simulink model "SRSModeState"  (R2018b)
settings: Solver=FixedStepDiscrete  StartTime=0.0  StopTime=10.0  FixedStep=0.01  RelTol=1e-3
undefined symbols (not defined in the file or in its folder): KeSMSuMdNums_Val, MdTp1, SrcReqTp1, SRSconvertArray_Val
libraries: RspLib x32
settings Model: Creator=sn2xws  LastModifiedBy=sn2xws
settings DataIOCC: SaveFormat=StructureWithTime
settings OptimizationCC: DefaultParameterBehavior=Inlined  EnhancedBackFolding=on  PassReuseOutputArgsAs=Individual arguments  ZeroExternalMemoryAtStartup=off  ZeroInternalMemoryAtStartup=off  OptimizeBlockOrder=speed  DifferentSizesBufferReuse=on  OptimizationCustomize=off
settings DebuggingCC: ParameterTunabilityLossMsg=error
settings ModelReferenceCC: ModelReferenceNumInstancesAllowed=Single
settings SFSimCC: MATLABDynamicMemAlloc=off
settings RTWCC: SystemTargetFile=autosar.tlc  GenCodeOnly=on  TemplateMakefile=ert_default_tmf  Description=AUTOSAR  GenerateReport=on  IncludeHyperlinkInReport=on  LaunchReport=on  GenerateTraceInfo=on  GenerateTraceReport=on  GenerateTraceReportSl=on  GenerateTraceReportSf=on  GenerateTraceReportEml=on  GenerateCodeMetricsReport=on
settings CodeAppCC: ForceParamTrailComments=on  IgnoreCustomStorageClasses=off  OperatorAnnotations=on  SimulinkDataObjDesc=on  SFDataObjDesc=on  InsertBlockDesc=on
settings STFCustomTargetCC: TargetLangStandard=C99 (ISO)  MultiwordLength=256  ParMdlRefBuildCompliant=on  CompOptLevelCompliant=on  IncludeMdlTerminateFcn=off  CombineOutputUpdateFcns=on  SuppressErrorStatus=on  ERTCustomFileBanners=on  SupportNonFinite=off  SupportComplex=off  SupportContinuousTime=off  SupportNonInlinedSFcns=off  RemoveResetFunc=on  MATLABClassNameForMDSCustomization=Simulink.SoftwareTarget.ERTCustomization  AutosarCompliant=on  UseToolchainInfoCompliant=on  LookupTableObjectStructAxisOrder=2,1,3,4,...  LUTObjectStructOrderEvenSpacing=Size,Table,Breakpoints  SystemTargetFile=autosar.tlc
settings ERTTargetCC: TargetLangStandard=C99 (ISO)  ConcurrentExecutionCompliant=off  IncludeMdlTerminateFcn=off  SuppressErrorStatus=on  SupportNonFinite=off  SupportComplex=off  ModelStepFunctionPrototypeControlCompliant=off  CPPClassGenCompliant=off  AutosarCompliant=on  LookupTableObjectStructAxisOrder=2,1,3,4,...  LUTObjectStructOrderEvenSpacing=Size,Table,Breakpoints  InlinedParameterPlacement=NonHierarchical  ERTCustomFileTemplate=example_file_process.tlc  ERTFilePackagingFormat=Compact

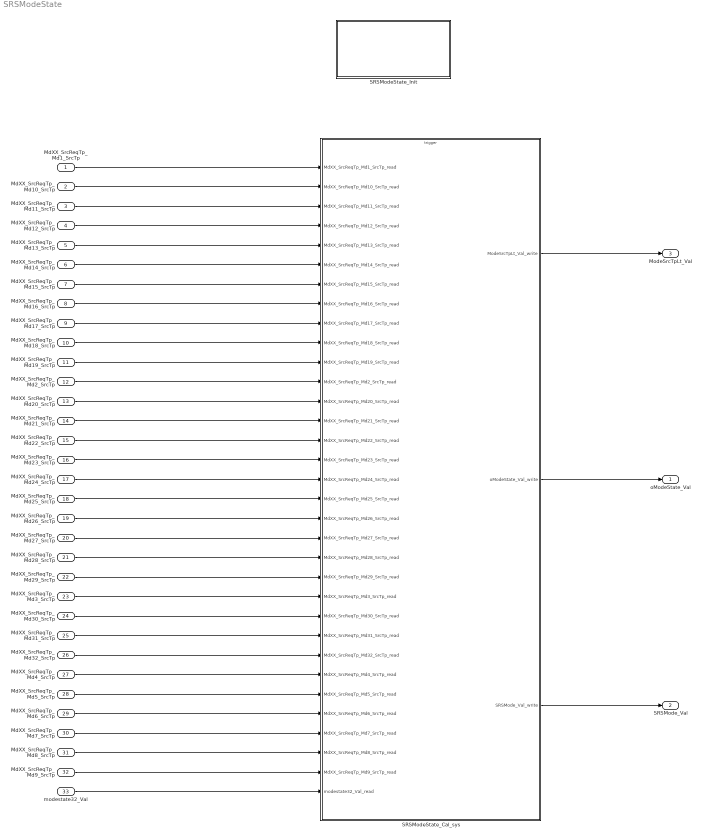
== system SRSModeState ==
  MdXX_SrcReqTp_Md1_SrcTp : Inport  OutDataTypeStr=Enum: SrcReqTp1  PortDimensions=1
  MdXX_SrcReqTp_Md10_SrcTp : Inport  Port=2  OutDataTypeStr=Enum: SrcReqTp1  PortDimensions=1
  MdXX_SrcReqTp_Md11_SrcTp : Inport  Port=3  OutDataTypeStr=Enum: SrcReqTp1  PortDimensions=1
  MdXX_SrcReqTp_Md12_SrcTp : Inport  Port=4  OutDataTypeStr=Enum: SrcReqTp1  PortDimensions=1
  MdXX_SrcReqTp_Md13_SrcTp : Inport  Port=5  OutDataTypeStr=Enum: SrcReqTp1  PortDimensions=1
  MdXX_SrcReqTp_Md14_SrcTp : Inport  Port=6  OutDataTypeStr=Enum: SrcReqTp1  PortDimensions=1
  MdXX_SrcReqTp_Md15_SrcTp : Inport  Port=7  OutDataTypeStr=Enum: SrcReqTp1  PortDimensions=1
  MdXX_SrcReqTp_Md16_SrcTp : Inport  Port=8  OutDataTypeStr=Enum: SrcReqTp1  PortDimensions=1
  MdXX_SrcReqTp_Md17_SrcTp : Inport  Port=9  OutDataTypeStr=Enum: SrcReqTp1  PortDimensions=1
  MdXX_SrcReqTp_Md18_SrcTp : Inport  Port=10  OutDataTypeStr=Enum: SrcReqTp1  PortDimensions=1
  MdXX_SrcReqTp_Md19_SrcTp : Inport  Port=11  OutDataTypeStr=Enum: SrcReqTp1  PortDimensions=1
  MdXX_SrcReqTp_Md2_SrcTp : Inport  Port=12  OutDataTypeStr=Enum: SrcReqTp1  PortDimensions=1
  MdXX_SrcReqTp_Md20_SrcTp : Inport  Port=13  OutDataTypeStr=Enum: SrcReqTp1  PortDimensions=1
  MdXX_SrcReqTp_Md21_SrcTp : Inport  Port=14  OutDataTypeStr=Enum: SrcReqTp1  PortDimensions=1
  MdXX_SrcReqTp_Md22_SrcTp : Inport  Port=15  OutDataTypeStr=Enum: SrcReqTp1  PortDimensions=1
  MdXX_SrcReqTp_Md23_SrcTp : Inport  Port=16  OutDataTypeStr=Enum: SrcReqTp1  PortDimensions=1
  MdXX_SrcReqTp_Md24_SrcTp : Inport  Port=17  OutDataTypeStr=Enum: SrcReqTp1  PortDimensions=1
  MdXX_SrcReqTp_Md25_SrcTp : Inport  Port=18  OutDataTypeStr=Enum: SrcReqTp1  PortDimensions=1
  MdXX_SrcReqTp_Md26_SrcTp : Inport  Port=19  OutDataTypeStr=Enum: SrcReqTp1  PortDimensions=1
  MdXX_SrcReqTp_Md27_SrcTp : Inport  Port=20  OutDataTypeStr=Enum: SrcReqTp1  PortDimensions=1
  MdXX_SrcReqTp_Md28_SrcTp : Inport  Port=21  OutDataTypeStr=Enum: SrcReqTp1  PortDimensions=1
  MdXX_SrcReqTp_Md29_SrcTp : Inport  Port=22  OutDataTypeStr=Enum: SrcReqTp1  PortDimensions=1
  MdXX_SrcReqTp_Md3_SrcTp : Inport  Port=23  OutDataTypeStr=Enum: SrcReqTp1  PortDimensions=1
  MdXX_SrcReqTp_Md30_SrcTp : Inport  Port=24  OutDataTypeStr=Enum: SrcReqTp1  PortDimensions=1
  MdXX_SrcReqTp_Md31_SrcTp : Inport  Port=25  OutDataTypeStr=Enum: SrcReqTp1  PortDimensions=1
  MdXX_SrcReqTp_Md32_SrcTp : Inport  Port=26  OutDataTypeStr=Enum: SrcReqTp1  PortDimensions=1
  MdXX_SrcReqTp_Md4_SrcTp : Inport  Port=27  OutDataTypeStr=Enum: SrcReqTp1  PortDimensions=1
  MdXX_SrcReqTp_Md5_SrcTp : Inport  Port=28  OutDataTypeStr=Enum: SrcReqTp1  PortDimensions=1
  MdXX_SrcReqTp_Md6_SrcTp : Inport  Port=29  OutDataTypeStr=Enum: SrcReqTp1  PortDimensions=1
  MdXX_SrcReqTp_Md7_SrcTp : Inport  Port=30  OutDataTypeStr=Enum: SrcReqTp1  PortDimensions=1
  MdXX_SrcReqTp_Md8_SrcTp : Inport  Port=31  OutDataTypeStr=Enum: SrcReqTp1  PortDimensions=1
  MdXX_SrcReqTp_Md9_SrcTp : Inport  Port=32  OutDataTypeStr=Enum: SrcReqTp1  PortDimensions=1
  modestate32_Val : Inport  Port=33  OutDataTypeStr=uint32  PortDimensions=1
  SRSModeState_Cal_sys : Subsystem
  SRSModeState_Init : Subsystem
  oModeState_Val : Outport  OutDataTypeStr=Enum: MdTp1  PortDimensions=1
  SRSMode_Val : Outport  Port=2  OutDataTypeStr=Enum: SRSCurMode2  PortDimensions=1
  ModeSrcTpLt_Val : Outport  Port=3  OutDataTypeStr=Enum: SrcReqTp1  PortDimensions=1
  wires:
  MdXX_SrcReqTp_Md1_SrcTp/1 -> SRSModeState_Cal_sys/1(MdXX_SrcReqTp_Md1_SrcTp_read)
  MdXX_SrcReqTp_Md10_SrcTp/1 -> SRSModeState_Cal_sys/2(MdXX_SrcReqTp_Md10_SrcTp_read)
  MdXX_SrcReqTp_Md11_SrcTp/1 -> SRSModeState_Cal_sys/3(MdXX_SrcReqTp_Md11_SrcTp_read)
  MdXX_SrcReqTp_Md12_SrcTp/1 -> SRSModeState_Cal_sys/4(MdXX_SrcReqTp_Md12_SrcTp_read)
  MdXX_SrcReqTp_Md13_SrcTp/1 -> SRSModeState_Cal_sys/5(MdXX_SrcReqTp_Md13_SrcTp_read)
  MdXX_SrcReqTp_Md14_SrcTp/1 -> SRSModeState_Cal_sys/6(MdXX_SrcReqTp_Md14_SrcTp_read)
  MdXX_SrcReqTp_Md15_SrcTp/1 -> SRSModeState_Cal_sys/7(MdXX_SrcReqTp_Md15_SrcTp_read)
  MdXX_SrcReqTp_Md16_SrcTp/1 -> SRSModeState_Cal_sys/8(MdXX_SrcReqTp_Md16_SrcTp_read)
  MdXX_SrcReqTp_Md17_SrcTp/1 -> SRSModeState_Cal_sys/9(MdXX_SrcReqTp_Md17_SrcTp_read)
  MdXX_SrcReqTp_Md18_SrcTp/1 -> SRSModeState_Cal_sys/10(MdXX_SrcReqTp_Md18_SrcTp_read)
  MdXX_SrcReqTp_Md19_SrcTp/1 -> SRSModeState_Cal_sys/11(MdXX_SrcReqTp_Md19_SrcTp_read)
  MdXX_SrcReqTp_Md2_SrcTp/1 -> SRSModeState_Cal_sys/12(MdXX_SrcReqTp_Md2_SrcTp_read)
  MdXX_SrcReqTp_Md20_SrcTp/1 -> SRSModeState_Cal_sys/13(MdXX_SrcReqTp_Md20_SrcTp_read)
  MdXX_SrcReqTp_Md21_SrcTp/1 -> SRSModeState_Cal_sys/14(MdXX_SrcReqTp_Md21_SrcTp_read)
  MdXX_SrcReqTp_Md22_SrcTp/1 -> SRSModeState_Cal_sys/15(MdXX_SrcReqTp_Md22_SrcTp_read)
  MdXX_SrcReqTp_Md23_SrcTp/1 -> SRSModeState_Cal_sys/16(MdXX_SrcReqTp_Md23_SrcTp_read)
  MdXX_SrcReqTp_Md24_SrcTp/1 -> SRSModeState_Cal_sys/17(MdXX_SrcReqTp_Md24_SrcTp_read)
  MdXX_SrcReqTp_Md25_SrcTp/1 -> SRSModeState_Cal_sys/18(MdXX_SrcReqTp_Md25_SrcTp_read)
  MdXX_SrcReqTp_Md26_SrcTp/1 -> SRSModeState_Cal_sys/19(MdXX_SrcReqTp_Md26_SrcTp_read)
  MdXX_SrcReqTp_Md27_SrcTp/1 -> SRSModeState_Cal_sys/20(MdXX_SrcReqTp_Md27_SrcTp_read)
  MdXX_SrcReqTp_Md28_SrcTp/1 -> SRSModeState_Cal_sys/21(MdXX_SrcReqTp_Md28_SrcTp_read)
  MdXX_SrcReqTp_Md29_SrcTp/1 -> SRSModeState_Cal_sys/22(MdXX_SrcReqTp_Md29_SrcTp_read)
  MdXX_SrcReqTp_Md3_SrcTp/1 -> SRSModeState_Cal_sys/23(MdXX_SrcReqTp_Md3_SrcTp_read)
  MdXX_SrcReqTp_Md30_SrcTp/1 -> SRSModeState_Cal_sys/24(MdXX_SrcReqTp_Md30_SrcTp_read)
  MdXX_SrcReqTp_Md31_SrcTp/1 -> SRSModeState_Cal_sys/25(MdXX_SrcReqTp_Md31_SrcTp_read)
  MdXX_SrcReqTp_Md32_SrcTp/1 -> SRSModeState_Cal_sys/26(MdXX_SrcReqTp_Md32_SrcTp_read)
  MdXX_SrcReqTp_Md4_SrcTp/1 -> SRSModeState_Cal_sys/27(MdXX_SrcReqTp_Md4_SrcTp_read)
  MdXX_SrcReqTp_Md5_SrcTp/1 -> SRSModeState_Cal_sys/28(MdXX_SrcReqTp_Md5_SrcTp_read)
  MdXX_SrcReqTp_Md6_SrcTp/1 -> SRSModeState_Cal_sys/29(MdXX_SrcReqTp_Md6_SrcTp_read)
  MdXX_SrcReqTp_Md7_SrcTp/1 -> SRSModeState_Cal_sys/30(MdXX_SrcReqTp_Md7_SrcTp_read)
  MdXX_SrcReqTp_Md8_SrcTp/1 -> SRSModeState_Cal_sys/31(MdXX_SrcReqTp_Md8_SrcTp_read)
  MdXX_SrcReqTp_Md9_SrcTp/1 -> SRSModeState_Cal_sys/32(MdXX_SrcReqTp_Md9_SrcTp_read)
  modestate32_Val/1 -> SRSModeState_Cal_sys/33(modestate32_Val_read)
  SRSModeState_Cal_sys/1(ModeSrcTpLt_Val_write) -> ModeSrcTpLt_Val/1
  SRSModeState_Cal_sys/3(SRSMode_Val_write) -> SRSMode_Val/1
  SRSModeState_Cal_sys/2(oModeState_Val_write) -> oModeState_Val/1

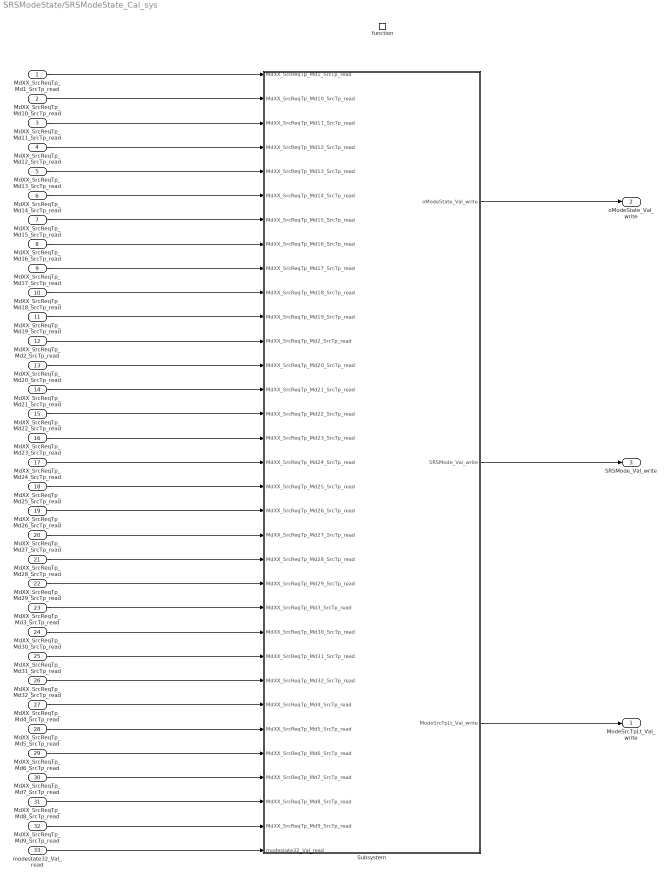
== system SRSModeState/SRSModeState_Cal_sys ==
  MdXX_SrcReqTp_Md1_SrcTp_read : Inport
  MdXX_SrcReqTp_Md10_SrcTp_read : Inport  Port=2
  MdXX_SrcReqTp_Md11_SrcTp_read : Inport  Port=3
  MdXX_SrcReqTp_Md12_SrcTp_read : Inport  Port=4
  MdXX_SrcReqTp_Md13_SrcTp_read : Inport  Port=5
  MdXX_SrcReqTp_Md14_SrcTp_read : Inport  Port=6
  MdXX_SrcReqTp_Md15_SrcTp_read : Inport  Port=7
  MdXX_SrcReqTp_Md16_SrcTp_read : Inport  Port=8
  MdXX_SrcReqTp_Md17_SrcTp_read : Inport  Port=9
  MdXX_SrcReqTp_Md18_SrcTp_read : Inport  Port=10
  MdXX_SrcReqTp_Md19_SrcTp_read : Inport  Port=11
  MdXX_SrcReqTp_Md2_SrcTp_read : Inport  Port=12
  MdXX_SrcReqTp_Md20_SrcTp_read : Inport  Port=13
  MdXX_SrcReqTp_Md21_SrcTp_read : Inport  Port=14
  MdXX_SrcReqTp_Md22_SrcTp_read : Inport  Port=15
  MdXX_SrcReqTp_Md23_SrcTp_read : Inport  Port=16
  MdXX_SrcReqTp_Md24_SrcTp_read : Inport  Port=17
  MdXX_SrcReqTp_Md25_SrcTp_read : Inport  Port=18
  MdXX_SrcReqTp_Md26_SrcTp_read : Inport  Port=19
  MdXX_SrcReqTp_Md27_SrcTp_read : Inport  Port=20
  MdXX_SrcReqTp_Md28_SrcTp_read : Inport  Port=21
  MdXX_SrcReqTp_Md29_SrcTp_read : Inport  Port=22
  MdXX_SrcReqTp_Md3_SrcTp_read : Inport  Port=23
  MdXX_SrcReqTp_Md30_SrcTp_read : Inport  Port=24
  MdXX_SrcReqTp_Md31_SrcTp_read : Inport  Port=25
  MdXX_SrcReqTp_Md32_SrcTp_read : Inport  Port=26
  MdXX_SrcReqTp_Md4_SrcTp_read : Inport  Port=27
  MdXX_SrcReqTp_Md5_SrcTp_read : Inport  Port=28
  MdXX_SrcReqTp_Md6_SrcTp_read : Inport  Port=29
  MdXX_SrcReqTp_Md7_SrcTp_read : Inport  Port=30
  MdXX_SrcReqTp_Md8_SrcTp_read : Inport  Port=31
  MdXX_SrcReqTp_Md9_SrcTp_read : Inport  Port=32
  modestate32_Val_read : Inport  Port=33
  function : TriggerPort  TriggerType=function-call  IsSimulinkFunction=on  FunctionName=SRSModeState_Cal  VariantControl=(inherit)
  Subsystem : Subsystem
  ModeSrcTpLt_Val_write : Outport
      settings: EnsureOutportIsVirtual=on
  oModeState_Val_write : Outport  Port=2
      settings: EnsureOutportIsVirtual=on
  SRSMode_Val_write : Outport  Port=3
      settings: EnsureOutportIsVirtual=on
  wires:
  MdXX_SrcReqTp_Md12_SrcTp_read/1 -> Subsystem/4(MdXX_SrcReqTp_Md12_SrcTp_read)
  MdXX_SrcReqTp_Md13_SrcTp_read/1 -> Subsystem/5(MdXX_SrcReqTp_Md13_SrcTp_read)
  MdXX_SrcReqTp_Md1_SrcTp_read/1 -> Subsystem/1(MdXX_SrcReqTp_Md1_SrcTp_read)
  MdXX_SrcReqTp_Md10_SrcTp_read/1 -> Subsystem/2(MdXX_SrcReqTp_Md10_SrcTp_read)
  MdXX_SrcReqTp_Md11_SrcTp_read/1 -> Subsystem/3(MdXX_SrcReqTp_Md11_SrcTp_read)
  MdXX_SrcReqTp_Md14_SrcTp_read/1 -> Subsystem/6(MdXX_SrcReqTp_Md14_SrcTp_read)
  MdXX_SrcReqTp_Md15_SrcTp_read/1 -> Subsystem/7(MdXX_SrcReqTp_Md15_SrcTp_read)
  MdXX_SrcReqTp_Md16_SrcTp_read/1 -> Subsystem/8(MdXX_SrcReqTp_Md16_SrcTp_read)
  MdXX_SrcReqTp_Md17_SrcTp_read/1 -> Subsystem/9(MdXX_SrcReqTp_Md17_SrcTp_read)
  MdXX_SrcReqTp_Md18_SrcTp_read/1 -> Subsystem/10(MdXX_SrcReqTp_Md18_SrcTp_read)
  MdXX_SrcReqTp_Md19_SrcTp_read/1 -> Subsystem/11(MdXX_SrcReqTp_Md19_SrcTp_read)
  MdXX_SrcReqTp_Md2_SrcTp_read/1 -> Subsystem/12(MdXX_SrcReqTp_Md2_SrcTp_read)
  MdXX_SrcReqTp_Md20_SrcTp_read/1 -> Subsystem/13(MdXX_SrcReqTp_Md20_SrcTp_read)
  MdXX_SrcReqTp_Md21_SrcTp_read/1 -> Subsystem/14(MdXX_SrcReqTp_Md21_SrcTp_read)
  MdXX_SrcReqTp_Md22_SrcTp_read/1 -> Subsystem/15(MdXX_SrcReqTp_Md22_SrcTp_read)
  MdXX_SrcReqTp_Md23_SrcTp_read/1 -> Subsystem/16(MdXX_SrcReqTp_Md23_SrcTp_read)
  MdXX_SrcReqTp_Md24_SrcTp_read/1 -> Subsystem/17(MdXX_SrcReqTp_Md24_SrcTp_read)
  MdXX_SrcReqTp_Md25_SrcTp_read/1 -> Subsystem/18(MdXX_SrcReqTp_Md25_SrcTp_read)
  MdXX_SrcReqTp_Md26_SrcTp_read/1 -> Subsystem/19(MdXX_SrcReqTp_Md26_SrcTp_read)
  MdXX_SrcReqTp_Md27_SrcTp_read/1 -> Subsystem/20(MdXX_SrcReqTp_Md27_SrcTp_read)
  MdXX_SrcReqTp_Md28_SrcTp_read/1 -> Subsystem/21(MdXX_SrcReqTp_Md28_SrcTp_read)
  MdXX_SrcReqTp_Md29_SrcTp_read/1 -> Subsystem/22(MdXX_SrcReqTp_Md29_SrcTp_read)
  MdXX_SrcReqTp_Md3_SrcTp_read/1 -> Subsystem/23(MdXX_SrcReqTp_Md3_SrcTp_read)
  MdXX_SrcReqTp_Md30_SrcTp_read/1 -> Subsystem/24(MdXX_SrcReqTp_Md30_SrcTp_read)
  MdXX_SrcReqTp_Md31_SrcTp_read/1 -> Subsystem/25(MdXX_SrcReqTp_Md31_SrcTp_read)
  MdXX_SrcReqTp_Md32_SrcTp_read/1 -> Subsystem/26(MdXX_SrcReqTp_Md32_SrcTp_read)
  MdXX_SrcReqTp_Md4_SrcTp_read/1 -> Subsystem/27(MdXX_SrcReqTp_Md4_SrcTp_read)
  MdXX_SrcReqTp_Md5_SrcTp_read/1 -> Subsystem/28(MdXX_SrcReqTp_Md5_SrcTp_read)
  MdXX_SrcReqTp_Md6_SrcTp_read/1 -> Subsystem/29(MdXX_SrcReqTp_Md6_SrcTp_read)
  MdXX_SrcReqTp_Md7_SrcTp_read/1 -> Subsystem/30(MdXX_SrcReqTp_Md7_SrcTp_read)
  MdXX_SrcReqTp_Md8_SrcTp_read/1 -> Subsystem/31(MdXX_SrcReqTp_Md8_SrcTp_read)
  MdXX_SrcReqTp_Md9_SrcTp_read/1 -> Subsystem/32(MdXX_SrcReqTp_Md9_SrcTp_read)
  modestate32_Val_read/1 -> Subsystem/33(modestate32_Val_read)
  Subsystem/1(oModeState_Val_write) -> oModeState_Val_write/1
  Subsystem/2(SRSMode_Val_write) -> SRSMode_Val_write/1
  Subsystem/3(ModeSrcTpLt_Val_write) -> ModeSrcTpLt_Val_write/1

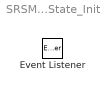
== system SRSModeState/SRSModeState_Init ==
  Event Listener : EventListener  EventName=reset

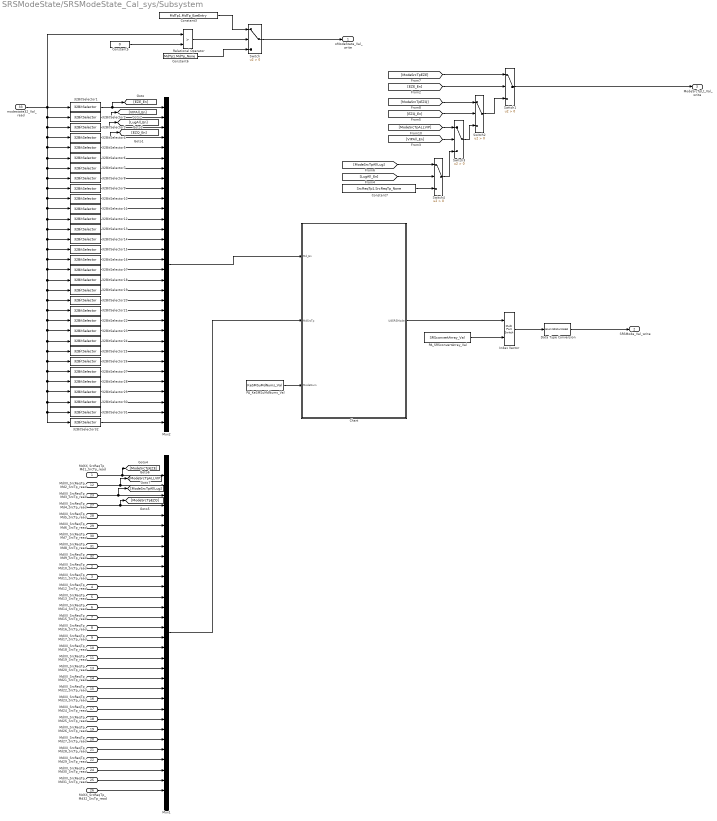
== system SRSModeState/SRSModeState_Cal_sys/Subsystem ==
  MdXX_SrcReqTp_Md1_SrcTp_read : Inport
  MdXX_SrcReqTp_Md10_SrcTp_read : Inport  Port=2
  MdXX_SrcReqTp_Md11_SrcTp_read : Inport  Port=3
  MdXX_SrcReqTp_Md12_SrcTp_read : Inport  Port=4
  MdXX_SrcReqTp_Md13_SrcTp_read : Inport  Port=5
  MdXX_SrcReqTp_Md14_SrcTp_read : Inport  Port=6
  MdXX_SrcReqTp_Md15_SrcTp_read : Inport  Port=7
  MdXX_SrcReqTp_Md16_SrcTp_read : Inport  Port=8
  MdXX_SrcReqTp_Md17_SrcTp_read : Inport  Port=9
  MdXX_SrcReqTp_Md18_SrcTp_read : Inport  Port=10
  MdXX_SrcReqTp_Md19_SrcTp_read : Inport  Port=11
  MdXX_SrcReqTp_Md2_SrcTp_read : Inport  Port=12
  MdXX_SrcReqTp_Md20_SrcTp_read : Inport  Port=13
  MdXX_SrcReqTp_Md21_SrcTp_read : Inport  Port=14
  MdXX_SrcReqTp_Md22_SrcTp_read : Inport  Port=15
  MdXX_SrcReqTp_Md23_SrcTp_read : Inport  Port=16
  MdXX_SrcReqTp_Md24_SrcTp_read : Inport  Port=17
  MdXX_SrcReqTp_Md25_SrcTp_read : Inport  Port=18
  MdXX_SrcReqTp_Md26_SrcTp_read : Inport  Port=19
  MdXX_SrcReqTp_Md27_SrcTp_read : Inport  Port=20
  MdXX_SrcReqTp_Md28_SrcTp_read : Inport  Port=21
  MdXX_SrcReqTp_Md29_SrcTp_read : Inport  Port=22
  MdXX_SrcReqTp_Md3_SrcTp_read : Inport  Port=23
  MdXX_SrcReqTp_Md30_SrcTp_read : Inport  Port=24
  MdXX_SrcReqTp_Md31_SrcTp_read : Inport  Port=25
  MdXX_SrcReqTp_Md32_SrcTp_read : Inport  Port=26
  MdXX_SrcReqTp_Md4_SrcTp_read : Inport  Port=27
  MdXX_SrcReqTp_Md5_SrcTp_read : Inport  Port=28
  MdXX_SrcReqTp_Md6_SrcTp_read : Inport  Port=29
  MdXX_SrcReqTp_Md7_SrcTp_read : Inport  Port=30
  MdXX_SrcReqTp_Md8_SrcTp_read : Inport  Port=31
  MdXX_SrcReqTp_Md9_SrcTp_read : Inport  Port=32
  modestate32_Val_read : Inport  Port=33
  32BitSelector1 : RspLib/32BitSelector  BitNum=0
  32BitSelector10 : RspLib/32BitSelector  BitNum=9
  32BitSelector11 : RspLib/32BitSelector  BitNum=10
  32BitSelector12 : RspLib/32BitSelector  BitNum=11
  32BitSelector13 : RspLib/32BitSelector  BitNum=12
  32BitSelector14 : RspLib/32BitSelector  BitNum=13
  32BitSelector15 : RspLib/32BitSelector  BitNum=14
  32BitSelector16 : RspLib/32BitSelector  BitNum=15
  32BitSelector17 : RspLib/32BitSelector  BitNum=16
  32BitSelector18 : RspLib/32BitSelector  BitNum=17
  32BitSelector19 : RspLib/32BitSelector  BitNum=18
  32BitSelector2 : RspLib/32BitSelector  BitNum=1
  32BitSelector20 : RspLib/32BitSelector  BitNum=19
  32BitSelector21 : RspLib/32BitSelector  BitNum=20
  32BitSelector22 : RspLib/32BitSelector  BitNum=21
  32BitSelector23 : RspLib/32BitSelector  BitNum=22
  32BitSelector24 : RspLib/32BitSelector  BitNum=23
  32BitSelector25 : RspLib/32BitSelector  BitNum=24
  32BitSelector26 : RspLib/32BitSelector  BitNum=25
  32BitSelector27 : RspLib/32BitSelector  BitNum=26
  32BitSelector28 : RspLib/32BitSelector  BitNum=27
  32BitSelector29 : RspLib/32BitSelector  BitNum=28
  32BitSelector3 : RspLib/32BitSelector  BitNum=2
  32BitSelector30 : RspLib/32BitSelector  BitNum=29
  32BitSelector31 : RspLib/32BitSelector  BitNum=30
  32BitSelector32 : RspLib/32BitSelector  BitNum=31
  32BitSelector4 : RspLib/32BitSelector  BitNum=3
  32BitSelector5 : RspLib/32BitSelector  BitNum=4
  32BitSelector6 : RspLib/32BitSelector  BitNum=5
  32BitSelector7 : RspLib/32BitSelector  BitNum=6
  32BitSelector8 : RspLib/32BitSelector  BitNum=7
  32BitSelector9 : RspLib/32BitSelector  BitNum=8
  Chart : Stateflow chart  TreatAsAtomicUnit=on
  Constant3 : Constant  Value=MdTp1.MdTp_EzeEntry  OutDataTypeStr=Enum:MdTp1
  Constant5 : Constant  Value=0  OutDataTypeStr=uint32
  Constant6 : Constant  Value=MdTp1.MdTp_None  OutDataTypeStr=Enum:MdTp1
  Constant7 : Constant  Value=SrcReqTp1.SrcReqTp_None  OutDataTypeStr=Enum:SrcReqTp1
  Data Type Conversion : DataTypeConversion  OutDataTypeStr=Enum:SRSCurMode2
  Index Vector : MultiPortSwitch  DataPortOrder=Zero-based contiguous  Inputs=1  zeroidx=on
  Mux1 : Mux  Inputs=32
  Mux2 : Mux  Inputs=32
  PA_KeSMSuMdNums_Val : Constant  Value=KeSMSuMdNums_Val
  PA_SRSconvertArray_Val : Constant  Value=SRSconvertArray_Val
  Relational Operator : RelationalOperator  Operator=>  OutDataTypeStr=boolean  RndMeth=Simplest
  Switch{,1..4} (5 alike) : Switch  Criteria=u2 > Threshold
  oModeState_Val_write : Outport
      settings: EnsureOutportIsVirtual=on
  SRSMode_Val_write : Outport  Port=2
      settings: EnsureOutportIsVirtual=on
  ModeSrcTpLt_Val_write : Outport  Port=3
      settings: EnsureOutportIsVirtual=on
  wires:
  Switch/1 -> oModeState_Val_write/1
  Index Vector/1 -> Data Type Conversion/1
  Data Type Conversion/1 -> SRSMode_Val_write/1
  Mux2/1 -> Chart/1(Md_En)
  Chart/1(U8SRSMode) -> Index Vector/1
  Mux1/1 -> Chart/2(MdSrcTp)
  PA_SRSconvertArray_Val/1 -> Index Vector/2
  PA_KeSMSuMdNums_Val/1 -> Chart/3(ModeNum)
  MdXX_SrcReqTp_Md14_SrcTp_read/1 -> Mux1/14
  MdXX_SrcReqTp_Md10_SrcTp_read/1 -> Mux1/10
  MdXX_SrcReqTp_Md4_SrcTp_read/1 -> [ModeSrcTpEZQ], Mux1/4
  MdXX_SrcReqTp_Md11_SrcTp_read/1 -> Mux1/11
  MdXX_SrcReqTp_Md15_SrcTp_read/1 -> Mux1/15
  MdXX_SrcReqTp_Md3_SrcTp_read/1 -> [ModeSrcTpAllLug], Mux1/3
  MdXX_SrcReqTp_Md12_SrcTp_read/1 -> Mux1/12
  MdXX_SrcReqTp_Md13_SrcTp_read/1 -> Mux1/13
  MdXX_SrcReqTp_Md9_SrcTp_read/1 -> Mux1/9
  MdXX_SrcReqTp_Md8_SrcTp_read/1 -> Mux1/8
  MdXX_SrcReqTp_Md7_SrcTp_read/1 -> Mux1/7
  MdXX_SrcReqTp_Md2_SrcTp_read/1 -> [ModeSrcTpALLVIP], Mux1/2
  MdXX_SrcReqTp_Md18_SrcTp_read/1 -> Mux1/18
  MdXX_SrcReqTp_Md6_SrcTp_read/1 -> Mux1/6
  MdXX_SrcReqTp_Md1_SrcTp_read/1 -> [ModeSrcTpEZE], Mux1/1
  MdXX_SrcReqTp_Md19_SrcTp_read/1 -> Mux1/19
  MdXX_SrcReqTp_Md5_SrcTp_read/1 -> Mux1/5
  MdXX_SrcReqTp_Md20_SrcTp_read/1 -> Mux1/20
  MdXX_SrcReqTp_Md17_SrcTp_read/1 -> Mux1/17
  MdXX_SrcReqTp_Md16_SrcTp_read/1 -> Mux1/16
  32BitSelector1/1 -> [EZE_En], Mux2/1
  32BitSelector2/1 -> [VIPAll_En], Mux2/2
  32BitSelector3/1 -> [LugAll_En], Mux2/3
  32BitSelector4/1 -> Mux2/4, [EZQ_En]
  32BitSelector5/1 -> Mux2/5
  32BitSelector6/1 -> Mux2/6
  32BitSelector7/1 -> Mux2/7
  32BitSelector8/1 -> Mux2/8
  32BitSelector9/1 -> Mux2/9
  32BitSelector10/1 -> Mux2/10
  32BitSelector11/1 -> Mux2/11
  32BitSelector12/1 -> Mux2/12
  32BitSelector13/1 -> Mux2/13
  32BitSelector14/1 -> Mux2/14
  32BitSelector15/1 -> Mux2/15
  32BitSelector16/1 -> Mux2/16
  32BitSelector17/1 -> Mux2/17
  32BitSelector18/1 -> Mux2/18
  32BitSelector19/1 -> Mux2/19
  32BitSelector20/1 -> Mux2/20
  Constant3/1 -> Switch/1
  Constant5/1 -> Relational Operator/2
  Constant6/1 -> Switch/3
  Relational Operator/1 -> Switch/2
  [EZE_En] -> Switch1/2
  [ModeSrcTpEZQ] -> Switch2/1
  [ModeSrcTpALLVIP] -> Switch3/1
  Switch1/1 -> ModeSrcTpLt_Val_write/1
  [VIPAll_En] -> Switch3/2
  Switch2/1 -> Switch1/3
  [LugAll_En] -> Switch4/2
  [ModeSrcTpEZE] -> Switch1/1
  [ModeSrcTpAllLug] -> Switch4/1
  Constant7/1 -> Switch4/3
  Switch3/1 -> Switch2/3
  [EZQ_En] -> Switch2/2
  Switch4/1 -> Switch3/3
  32BitSelector21/1 -> Mux2/21
  32BitSelector22/1 -> Mux2/22
  32BitSelector23/1 -> Mux2/23
  32BitSelector24/1 -> Mux2/24
  32BitSelector25/1 -> Mux2/25
  32BitSelector26/1 -> Mux2/26
  modestate32_Val_read/1 -> Relational Operator/1, 32BitSelector20/1, 32BitSelector21/1, 32BitSelector32/1, 32BitSelector31/1, 32BitSelector30/1, 32BitSelector29/1, 32BitSelector28/1, 32BitSelector27/1, 32BitSelector26/1, 32BitSelector25/1, 32BitSelector24/1, 32BitSelector23/1, 32BitSelector22/1, 32BitSelector19/1, 32BitSelector18/1, 32BitSelector17/1, 32BitSelector16/1, 32BitSelector15/1, 32BitSelector14/1, 32BitSelector13/1, 32BitSelector12/1, 32BitSelector11/1, 32BitSelector10/1, 32BitSelector9/1, 32BitSelector8/1, 32BitSelector7/1, 32BitSelector6/1, 32BitSelector5/1, 32BitSelector4/1, 32BitSelector3/1, 32BitSelector2/1, 32BitSelector1/1
  MdXX_SrcReqTp_Md21_SrcTp_read/1 -> Mux1/21
  MdXX_SrcReqTp_Md22_SrcTp_read/1 -> Mux1/22
  MdXX_SrcReqTp_Md23_SrcTp_read/1 -> Mux1/23
  MdXX_SrcReqTp_Md24_SrcTp_read/1 -> Mux1/24
  MdXX_SrcReqTp_Md25_SrcTp_read/1 -> Mux1/25
  MdXX_SrcReqTp_Md26_SrcTp_read/1 -> Mux1/26
  32BitSelector27/1 -> Mux2/27
  32BitSelector28/1 -> Mux2/28
  32BitSelector29/1 -> Mux2/29
  32BitSelector30/1 -> Mux2/30
  32BitSelector31/1 -> Mux2/31
  32BitSelector32/1 -> Mux2/32
  MdXX_SrcReqTp_Md27_SrcTp_read/1 -> Mux1/27
  MdXX_SrcReqTp_Md28_SrcTp_read/1 -> Mux1/28
  MdXX_SrcReqTp_Md29_SrcTp_read/1 -> Mux1/29
  MdXX_SrcReqTp_Md30_SrcTp_read/1 -> Mux1/30
  MdXX_SrcReqTp_Md31_SrcTp_read/1 -> Mux1/31
  MdXX_SrcReqTp_Md32_SrcTp_read/1 -> Mux1/32

== stateflow chart SRSModeState/SRSModeState_Cal_sys/Subsystem/Chart ==
  (default) -> (junction 5) : {i=0;}
  (junction 7) -> (junction 10) [order 1] : [Md_En[i] ==1&&MdSrcTp[i] ==SrcReqTp1.SrcReqTp_SRS]
  (junction 5) -> (junction 7) [order 1] : [i<ModeNum]
  (junction 7) -> (junction 16) [order 2]
  (junction 10) -> (junction 12) : {
      | U8SRSMode=i+1;
      | }
  (junction 16) -> (junction 5) : {i=i+1;}
  (junction 5) -> (junction 14) [order 2] : {
      | U8SRSMode=0;
      | }
  (junction 12) -> (junction 14)
  (junction 14) -> (junction 20)
  data: i local uint8; Md_En input boolean size=32; MdSrcTp input Enum: SrcReqTp1 size=32; U8SRSMode output uint8; ModeNum input uint8
